simulink model "Exemple_notes"  (R2018a)
settings: Solver=VariableStepAuto  StartTime=0.0  StopTime=simTime  RelTol=1e-3
undefined symbols (not defined in the file): ramp
libraries: simulink x1
settings Model: Creator=chsira  LastModifiedBy=charl
settings SolverCC: MaxConsecutiveZCs=100
settings DebuggingCC: MaxConsecutiveZCsMsg=none  LibraryContextMissingDiagnostic=warning
settings SFSimCC: SimUseLocalCustomCode=on
settings RTWCC: RTWUseLocalCustomCode=on

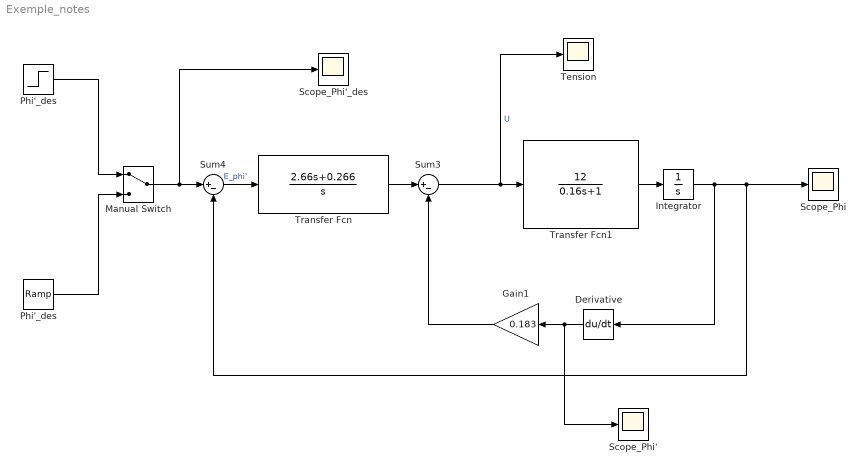
== system Exemple_notes ==
  Derivative : Derivative
  Gain1 : Gain  Gain=0.183
  Integrator : Integrator
  Manual Switch : ManualSwitch
  Phi'_des : simulink/Sources/Ramp  slope=ramp  start=0  InitialOutput=0
  "Phi'_des " : Step  Time=0  After=pi  SampleTime=0
  Scope_Phi : Scope
  Scope_Phi' : Scope
  Scope_Phi'_des : Scope
  Sum3 : Sum  Inputs=|+-
  Sum4 : Sum  Inputs=|+-
  Tension : Scope
  Transfer Fcn : TransferFcn  Numerator=[2.66 0.266]  Denominator=[1 0]
  Transfer Fcn1 : TransferFcn  Numerator=[12]  Denominator=[0.16 1]
  wires:
  Sum3/1 -> Transfer Fcn1/1, Tension/1  "U"
  Sum4/1 -> Transfer Fcn/1  "E_phi'"
  Gain1/1 -> Sum3/2
  Transfer Fcn/1 -> Sum3/1
  "Phi'_des "/1 -> Manual Switch/1
  Phi'_des/1 -> Manual Switch/2
  Transfer Fcn1/1 -> Integrator/1
  Derivative/1 -> Scope_Phi'/1, Gain1/1
  Integrator/1 -> Derivative/1, Scope_Phi/1, Sum4/2
  Manual Switch/1 -> Scope_Phi'_des/1, Sum4/1
